simulink model "PVarray_Grid_IncCondReg_det"  (Simulink 10.0)
settings: Solver=FixedStepDiscrete  StartTime=0.0  StopTime=3  RelTol=1e-3
PreLoadFcn:
  | Ts_Power=1e-6
  | Ts_Control=100e-6
undefined symbols (not defined in the file): D1, Delta, DiscIntNeverNeededParam, level, sigbuilder_block
libraries: powerlib x29, powerlib_extras x7, simulink x4
(part 2 of 2)

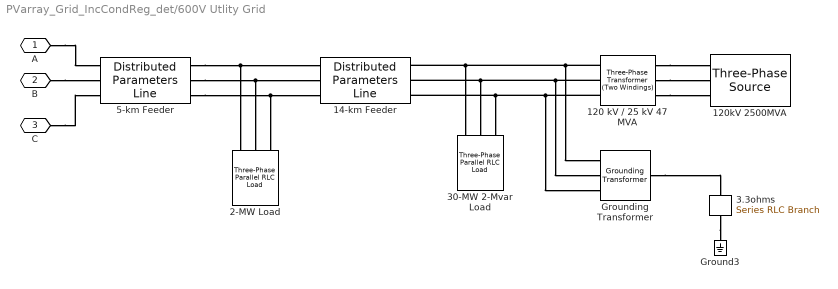
== system PVarray_Grid_IncCondReg_det/600V Utlity Grid ==
  120 kV / 25 kV 47 MVA : powerlib/Elements/Three-Phase Transformer (Two Windings)  Winding1Connection=Yg  Winding2Connection=Delta (D1)  CoreType=Three single-phase transformers  SetSaturation=off  Hysteresis=off  DataFile='basic_model'  SetInitialFlux=off  Measurements=None  UNITS=pu  NominalPower=[47e6 60 ]  Winding1="[ 120e3  0.08/30   0.08 ]"  Winding2="[ 25e3  0.08/30  0.08]"  Rm=500  Lm=500  L0=0.5  Saturation="[ 0,0  ;  0.005,1.2  ;  1.0,1.4 ]"  InitialFluxes=[ 0.8 , -0.8 , 0.7 ]  BreakLoop=off  DiscreteSolver=Trapezoidal iterative  DataType=off  TransfoNumber=0
      settings: SourceProductName=Simscape Electrical
  120kV 2500MVA : powerlib/Electrical Sources/Three-Phase Source  InternalConnection=Yg  VoltagePhases=off  Voltage=120e3  PhaseAngle=0  Voltage_phases=[25e3 25e3 25e3]/sqrt(3)  PhaseAngles_phases=[0 -120 +120]  Frequency=60  NonIdealSource=on  SpecifyImpedance=on  Resistance=0.8929  Inductance=16.58e-3  ShortCircuitLevel=2500e6  BaseVoltage=120e3  XRratio=7  BusType=swing  Pref=0  Qref=0  Prefabc=[10e3, 10e3, 10e3]  Qrefabc=[0, 0, 0]  Qmin=-inf  Qmax=inf
      settings: SourceProductName=Simscape Electrical
  14-km Feeder : powerlib/Elements/Distributed Parameters Line  Phases=3  Frequency=60  Resistance=[0.1153 0.413]  Inductance=[1.05e-3 3.32e-3]  Capacitance=[11.33e-009 5.01e-009]  Length=14  x1=[-5.8e-05 3.86893483226121e-09 0 0;-5.7e-05 3.86863781931287e-09 0 0;-5.6e-05 3.86834025654481e-09 0 0;-5.5e-05 3.86804214399933e-09 0 0;-5.4e-05 3.8677434817188e-09 0 0;-5.3e-05 3.86744426974566e-09 0 0;-5.2e-05 3.86714450812244e-09 0 0;-5.1e-05 3.86684419689175e-09 0 0;-5e-05 3.86654333609625e-09 0 0;-4.9e-05 3.86624192577872e-09 -3790.50088209685 -24060.9143986491;-4.8e-05 3.86593996598198e-09 -3781.42986192474 -24062.341673986;-4.7e-05 3.86563745674896e-09 -3772.35830432711 -24063.7655295274;-4.6e-05 3.86533439812265e-09 -3763.28621059323 -24065.1859650711;-4.5e-05 3.86503079014612e-09 -3754.21358201246 -24066.6029804152;-4.4e-05 3.86472663286251e-09 -3745.14041987422 -24068.0165753583;-4.3e-05 3.86442192631506e-09 -3736.06672546799 -24069.4267496995;-4.2e-05 3.86411667054707e-09 -3726.99250008337 -24070.8335032383;-4.1e-05 3.86381086560192e-09 -3717.91774500999 -24072.2368357749;-4e-05 3.86350451152308e-09 -3708.84246153758 -24073.6367471098;-3.9e-05 3.86319760835409e-09 -3699.76665095595 -24075.033237044;-3.8e-05 3.86289015613856e-09 -3690.69031455496 -24076.426305379;-3.7e-05 3.86258215492019e-09 -3681.61345362458 -24077.815951917;-3.6e-05 3.86227360474275e-09 -3672.53606945481 -24079.2021764603;-3.5e-05 3.8619645056501e-09 -3663.45816333577 -24080.584978812;-3.4e-05 3.86165485768617e-09 -3654.37973655762 -24081.9643587755;-3.3e-05 3.86134466089496e-09 -3645.30079041061 -24083.3403161549;-3.2e-05 3.86103391532056e-09 -3636.22132618506 -24084.7128507544;-3.1e-05 3.86072262100713e-09 -3627.14134517136 -24086.0819623792;-3e-05 3.86041077799891e-09 -3618.06084865999 -24087.4476508345;-2.9e-05 3.86009838634023e-09 -3608.97983794149 -24088.8099159263;-2.8e-05 3.85978544607549e-09 -3599.89831430646 -24090.168757461;-2.7e-05 3.85947195724915e-09 -3590.8162790456 -24091.5241752455;-2.6e-05 3.85915791990577e-09 -3581.73373344966 -24092.8761690871;-2.5e-05 3.85884333408999e-09 -3572.65067880949 -24094.2247387938;-2.4e-05 3.85852819984651e-09 -3563.56711641597 -24095.5698841737;-2.3e-05 3.85821251722012e-09 -3554.48304756009 -24096.9116050357;-2.2e-05 3.85789628625569e-09 -3545.39847353291 -24098.2499011893;-2.1e-05 3.85757950699816e-09 -3536.31339562553 -24099.5847724441;-2e-05 3.85726217949255e-09 -3527.22781512915 -24100.9162186104;-1.9e-05 3.85694430378396e-09 -3518.14173333503 -24102.244239499;-1.8e-05 3.85662587991757e-09 -3509.05515153452 -24103.5688349213;-1.7e-05 3.85630690793864e-09 -3499.96807101901 -24104.8900046888;-1.6e-05 3.85598738789248e-09 -3490.88049307998 -24106.2077486139;-1.5e-05 3.85566731982453e-09 -3481.79241900898 -24107.5220665093;-1.4e-05 3.85534670378026e-09 -3472.70385009763 -24108.8329581881;-1.3e-05 3.85502553980525e-09 -3463.61478763761 -24110.1404234641;-1.2e-05 3.85470382794513e-09 -3454.52523292069 -24111.4444621514;-1.1e-05 3.85438156824563e-09 -3445.43518723869 -24112.7450740648;-1e-05 3.85405876075255e-09 -3436.34465188351 -24114.0422590193;-9e-06 3.85373540551177e-09 -3427.25362814712 -24115.3360168307;-8e-06 3.85341150256924e-09 -3418.16211732156 -24116.626347315;-7e-06 3.853087051971e-09 -3409.07012069893 -24117.9132502888;-6e-06 3.85276205376316e-09 -3399.9776395714 -24119.1967255693;-5e-06 3.85243650799191e-09 -3390.88467523123 -24120.4767729741;-4e-06 3.85211041470352e-09 -3381.79122897072 -24121.7533923211;-3e-06 3.85178377394433e-09 -3372.69730208226 -24123.0265834291;-2e-06 3.85145658576076e-09 -3363.6028958583 -24124.296346117;-1e-06 3.85112885019932e-09 -3354.50801159135 -24125.5626802043]  x2=[-5.8e-05 4.13964869045981e-09 0 0;-5.7e-05 4.13926412209804e-09 0 0;-5.6e-05 4.13887896545453e-09 0 0;-5.5e-05 4.13849322058402e-09 0 0;-5.4e-05 4.13810688754132e-09 0 0;-5.3e-05 4.13771996638135e-09 0 0;-5.2e-05 4.1373324571591e-09 0 0;-5.1e-05 4.13694435992963e-09 0 0;-5e-05 4.13655567474811e-09 0 0;-4.9e-05 4.13616640166977e-09 -3379.33798533028 -24243.9018981742;-4.8e-05 4.13577654074994e-09 -3370.19800971541 -24245.1741557511;-4.7e-05 4.13538609204404e-09 -3361.05755512023 -24246.442967548;-4.6e-05 4.13499505560754e-09 -3351.91662284382 -24247.7083333847;-4.5e-05 4.13460343149603e-09 -3342.77521418531 -24248.9702530812;-4.4e-05 4.13421121976516e-09 -3333.63333044389 -24250.2287264583;-4.3e-05 4.13381842047068e-09 -3324.49097291882 -24251.4837533371;-4.2e-05 4.13342503366841e-09 -3315.34814290945 -24252.7353335391;-4.1e-05 4.13303105941426e-09 -3306.20484171517 -24253.9834668866;-4e-05 4.13263649776422e-09 -3297.06107063545 -24255.2281532022;-3.9e-05 4.13224134877437e-09 -3287.91683096981 -24256.4693923088;-3.8e-05 4.13184561250087e-09 -3278.77212401787 -24257.7071840303;-3.7e-05 4.13144928899996e-09 -3269.62695107929 -24258.9415281905;-3.6e-05 4.13105237832797e-09 -3260.4813134538 -24260.1724246142;-3.5e-05 4.13065488054131e-09 -3251.33521244121 -24261.3998731263;-3.4e-05 4.13025679569647e-09 -3242.18864934136 -24262.6238735524;-3.3e-05 4.12985812385002e-09 -3233.04162545421 -24263.8444257185;-3.2e-05 4.12945886505863e-09 -3223.89414207974 -24265.0615294512;-3.1e-05 4.12905901937905e-09 -3214.74620051801 -24266.2751845776;-3e-05 4.12865858686809e-09 -3205.59780206915 -24267.485390925;-2.9e-05 4.12825756758267e-09 -3196.44894803336 -24268.6921483216;-2.8e-05 4.12785596157979e-09 -3187.29963971088 -24269.8954565958;-2.7e-05 4.12745376891651e-09 -3178.14987840204 -24271.0953155766;-2.6e-05 4.12705098965e-09 -3168.99966540723 -24272.2917250934;-2.5e-05 4.12664762383751e-09 -3159.84900202689 -24273.4846849763;-2.4e-05 4.12624367153636e-09 -3150.69788956153 -24274.6741950557;-2.3e-05 4.12583913280396e-09 -3141.54632931174 -24275.8602551625;-2.2e-05 4.12543400769781e-09 -3132.39432257816 -24277.0428651282;-2.1e-05 4.12502829627548e-09 -3123.24187066148 -24278.2220247846;-2e-05 4.12462199859463e-09 -3114.08897486248 -24279.3977339643;-1.9e-05 4.12421511471301e-09 -3104.93563648199 -24280.5699925001;-1.8e-05 4.12380764468845e-09 -3095.7818568209 -24281.7388002254;-1.7e-05 4.12339958857886e-09 -3086.62763718016 -24282.904156974;-1.6e-05 4.12299094644222e-09 -3077.47297886081 -24284.0660625805;-1.5e-05 4.12258171833662e-09 -3068.3178831639 -24285.2245168796;-1.4e-05 4.12217190432022e-09 -3059.1623513906 -24286.3795197066;-1.3e-05 4.12176150445126e-09 -3050.00638484211 -24287.5310708975;-1.2e-05 4.12135051878806e-09 -3040.84998481968 -24288.6791702886;-1.1e-05 4.12093894738905e-09 -3031.69315262466 -24289.8238177168;-1e-05 4.1205267903127e-09 -3022.53588955843 -24290.9650130192;-9e-06 4.12011404761761e-09 -3013.37819692244 -24292.1027560338;-8e-06 4.11970071936242e-09 -3004.2200760182 -24293.2370465988;-7e-06 4.11928680560588e-09 -2995.0615281473 -24294.3678845531;-6e-06 4.11887230640683e-09 -2985.90255461135 -24295.4952697358;-5e-06 4.11845722182416e-09 -2976.74315671207 -24296.6192019869;-4e-06 4.11804155191686e-09 -2967.58333575119 -24297.7396811465;-3e-06 4.11762529674403e-09 -2958.42309303054 -24298.8567070555;-2e-06 4.11720845636481e-09 -2949.26242985199 -24299.970279555;-1e-06 4.11679103083845e-09 -2940.10134751747 -24301.0803984868]  x3=[-5.8e-05 2.1249422545882e-11 0 0;-5.7e-05 2.12530209427396e-11 0 0;-5.6e-05 2.1256616319069e-11 0 0;-5.5e-05 2.12602086743592e-11 0 0;-5.4e-05 2.12637980080996e-11 0 0;-5.3e-05 2.126738431978e-11 0 0;-5.2e-05 2.12709676088909e-11 0 0;-5.1e-05 2.12745478749228e-11 0 0;-5e-05 2.12781251173671e-11 0 0;-4.9e-05 2.12816993357152e-11 -23.610210034622 -155.666879550872;-4.8e-05 2.12852705294593e-11 -23.5515233272188 -155.675769328281;-4.7e-05 2.12888386980917e-11 -23.4928332726189 -155.684636980691;-4.6e-05 2.12924038411053e-11 -23.4341398791635 -155.693482506843;-4.5e-05 2.12959659579935e-11 -23.3754431551942 -155.702305905478;-4.4e-05 2.129952504825e-11 -23.3167431090532 -155.711107175343;-4.3e-05 2.1303081111369e-11 -23.2580397490829 -155.719886315187;-4.2e-05 2.13066341468451e-11 -23.1993330836265 -155.728643323763;-4.1e-05 2.13101841541732e-11 -23.1406231210274 -155.737378199825;-4e-05 2.1313731132849e-11 -23.0819098696298 -155.746090942133;-3.9e-05 2.13172750823682e-11 -23.023193337778 -155.754781549447;-3.8e-05 2.13208160022272e-11 -22.9644735338169 -155.763450020534;-3.7e-05 2.13243538919228e-11 -22.9057504660921 -155.772096354161;-3.6e-05 2.13278887509522e-11 -22.8470241429492 -155.780720549098;-3.5e-05 2.13314205788128e-11 -22.7882945727347 -155.789322604122;-3.4e-05 2.13349493750029e-11 -22.7295617637953 -155.797902518008;-3.3e-05 2.13384751390209e-11 -22.6708257244783 -155.806460289537;-3.2e-05 2.13419978703657e-11 -22.6120864631313 -155.814995917494;-3.1e-05 2.13455175685366e-11 -22.5533439881026 -155.823509400665;-3e-05 2.13490342330335e-11 -22.4945983077407 -155.83200073784;-2.9e-05 2.13525478633564e-11 -22.4358494303947 -155.840469927813;-2.8e-05 2.13560584590061e-11 -22.3770973644142 -155.848916969379;-2.7e-05 2.13595660194836e-11 -22.318342118149 -155.857341861338;-2.6e-05 2.13630705442905e-11 -22.2595836999498 -155.865744602493;-2.5e-05 2.13665720329285e-11 -22.2008221181672 -155.87412519165;-2.4e-05 2.13700704849002e-11 -22.1420573811527 -155.882483627618;-2.3e-05 2.13735658997083e-11 -22.0832894972581 -155.890819909208;-2.2e-05 2.1377058276856e-11 -22.0245184748355 -155.899134035236;-2.1e-05 2.13805476158469e-11 -21.9657443222377 -155.90742600452;-2e-05 2.13840339161853e-11 -21.9069670478177 -155.915695815882;-1.9e-05 2.13875171773755e-11 -21.8481866599292 -155.923943468146;-1.8e-05 2.13909973989225e-11 -21.789403166926 -155.932168960141;-1.7e-05 2.13944745803318e-11 -21.7306165771628 -155.940372290697;-1.6e-05 2.1397948721109e-11 -21.6718268989943 -155.948553458648;-1.5e-05 2.14014198207606e-11 -21.6130341407758 -155.956712462832;-1.4e-05 2.14048878787931e-11 -21.5542383108633 -155.964849302089;-1.3e-05 2.14083528947137e-11 -21.4954394176127 -155.972963975263;-1.2e-05 2.14118148680299e-11 -21.4366374693808 -155.981056481199;-1.1e-05 2.14152737982497e-11 -21.3778324745247 -155.98912681875;-1e-05 2.14187296848815e-11 -21.3190244414018 -155.997174986766;-9e-06 2.14221825274341e-11 -21.2602133783701 -156.005200984105;-8e-06 2.14256323254168e-11 -21.2013992937879 -156.013204809626;-7e-06 2.14290790783393e-11 -21.1425821960141 -156.02118646219;-6e-06 2.14325227857118e-11 -21.0837620934078 -156.029145940665;-5e-06 2.14359634470449e-11 -21.0249389943287 -156.037083243919;-4e-06 2.14394010618494e-11 -20.9661129071369 -156.044998370822;-3e-06 2.1442835629637e-11 -20.9072838401929 -156.052891320252;-2e-06 2.14462671499194e-11 -20.8484518018576 -156.060762091086;-1e-06 2.14496956222089e-11 -20.7896168004923 -156.068610682204]  x4=[-5.8e-05 -1.15723579337896e-11 0 0;-5.7e-05 -1.15764232992851e-11 0 0;-5.6e-05 -1.15804870195128e-11 0 0;-5.5e-05 -1.1584549093895e-11 0 0;-5.4e-05 -1.15886095218544e-11 0 0;-5.3e-05 -1.15926683028139e-11 0 0;-5.2e-05 -1.15967254361968e-11 0 0;-5.1e-05 -1.16007809214263e-11 0 0;-5e-05 -1.16048347579262e-11 0 0;-4.9e-05 -1.16088869451202e-11 -1.28892375629152 -2.16547060902535;-4.8e-05 -1.16129374824325e-11 -1.28810730153162 -2.16595636794147;-4.7e-05 -1.16169863692873e-11 -1.28729066370296 -2.16644181902688;-4.6e-05 -1.16210336051094e-11 -1.28647384292158 -2.16692696221259;-4.5e-05 -1.16250791893234e-11 -1.28565683930357 -2.16741179742966;-4.4e-05 -1.16291231213544e-11 -1.28483965296506 -2.16789632460917;-4.3e-05 -1.16331654006276e-11 -1.28402228402218 -2.16838054368227;-4.2e-05 -1.16372060265686e-11 -1.28320473259109 -2.16886445458013;-4.1e-05 -1.16412449986031e-11 -1.282386998788 -2.16934805723399;-4e-05 -1.1645282316157e-11 -1.28156908272911 -2.1698313515751;-3.9e-05 -1.16493179786567e-11 -1.28075098453068 -2.17031433753479;-3.8e-05 -1.16533519855284e-11 -1.27993270430896 -2.17079701504441;-3.7e-05 -1.1657384336199e-11 -1.27911424218027 -2.17127938403536;-3.6e-05 -1.16614150300952e-11 -1.27829559826092 -2.17176144443909;-3.5e-05 -1.16654440666443e-11 -1.27747677266725 -2.17224319618709;-3.4e-05 -1.16694714452737e-11 -1.27665776551564 -2.17272463921088;-3.3e-05 -1.16734971654109e-11 -1.2758385769225 -2.17320577344204;-3.2e-05 -1.16775212264838e-11 -1.27501920700423 -2.1736865988122;-3.1e-05 -1.16815436279205e-11 -1.27419965587731 -2.17416711525301;-3e-05 -1.16855643691493e-11 -1.27337992365819 -2.17464732269619;-2.9e-05 -1.16895834495989e-11 -1.27256001046339 -2.17512722107349;-2.8e-05 -1.16936008686979e-11 -1.27173991640944 -2.1756068103167;-2.7e-05 -1.16976166258755e-11 -1.27091964161288 -2.17608609035766;-2.6e-05 -1.17016307205609e-11 -1.27009918619029 -2.17656506112826;-2.5e-05 -1.17056431521835e-11 -1.26927855025828 -2.17704372256042;-2.4e-05 -1.17096539201733e-11 -1.26845773393349 -2.17752207458612;-2.3e-05 -1.171366302396e-11 -1.26763673733256 -2.17800011713737;-2.2e-05 -1.17176704629741e-11 -1.26681556057218 -2.17847785014623;-2.1e-05 -1.17216762366458e-11 -1.26599420376906 -2.1789552735448;-2e-05 -1.17256803444059e-11 -1.26517266703993 -2.17943238726523;-1.9e-05 -1.17296827856853e-11 -1.26435095050155 -2.17990919123972;-1.8e-05 -1.17336835599152e-11 -1.2635290542707 -2.18038568540049;-1.7e-05 -1.1737682666527e-11 -1.26270697846419 -2.18086186967984;-1.6e-05 -1.17416801049524e-11 -1.26188472319886 -2.18133774401007;-1.5e-05 -1.17456758746231e-11 -1.26106228859157 -2.18181330832356;-1.4e-05 -1.17496699749713e-11 -1.2602396747592 -2.18228856255273;-1.3e-05 -1.17536624054294e-11 -1.25941688181867 -2.18276350663002;-1.2e-05 -1.17576531654299e-11 -1.25859390988691 -2.18323814048793;-1.1e-05 -1.17616422544057e-11 -1.25777075908089 -2.18371246405902;-1e-05 -1.17656296717899e-11 -1.2569474295176 -2.18418647727587;-9e-06 -1.17696154170156e-11 -1.25612392131404 -2.1846601800711;-8e-06 -1.17735994895166e-11 -1.25530023458726 -2.18513357237741;-7e-06 -1.17775818887265e-11 -1.25447636945433 -2.18560665412749;-6e-06 -1.17815626140793e-11 -1.25365232603232 -2.18607942525414;-5e-06 -1.17855416650093e-11 -1.25282810443836 -2.18655188569014;-4e-06 -1.1789519040951e-11 -1.25200370478958 -2.18702403536835;-3e-06 -1.17934947413392e-11 -1.25117912720316 -2.18749587422168;-2e-06 -1.17974687656087e-11 -1.25035437179628 -2.18796740218306;-1e-06 -1.18014411131948e-11 -1.24952943868616 -2.18843861918547]  x5=5.70973484498186e-05  V1=ones(3,3)  V2=ones(3,3)  I1=ones(3,3)  I2=ones(3,3)  nHarmo=1  Measurements=None
      settings: SourceProductName=Simscape Electrical
  2-MW Load : powerlib/Elements/Three-Phase Parallel RLC Load  LConnTagsString=A|B|C  Configuration=Y (grounded)  NominalVoltage=25e3  Vabc=[1e3 1e3 1e3]  Vabcp=[1e3 1e3 1e3]  NominalFrequency=60  UnbalancedPower=off  ActivePower=2e6  InductivePower=0  CapacitivePower=0  Pabc=[10e3 9e3 11e3]  QLabc=[100 90 110]  QCabc=[100 90 110]  Pabcp=[10e3 9e3 11e3]  QLabcp=[100 90 110]  QCabcp=[100 90 110]  Measurements=None  LoadType=constant Z
      settings: SourceProductName=Simscape Electrical
  "3.3ohms " : powerlib/Elements/Series RLC Branch  LConnTagsString=__new0  RConnTagsString=__new0  BranchType=R  Resistance=3.3  Inductance=[]  SetiL0=off  InitialCurrent=0  Capacitance=[]  Setx0=off  InitialVoltage=0  Measurements=None
      settings: SourceProductName=Simscape Electrical
  30-MW 2-Mvar Load : powerlib/Elements/Three-Phase Parallel RLC Load  LConnTagsString=A|B|C  Configuration=Y (grounded)  NominalVoltage=25e3  Vabc=[1e3 1e3 1e3]  Vabcp=[1e3 1e3 1e3]  NominalFrequency=60  UnbalancedPower=off  ActivePower=30e6  InductivePower=2e6  CapacitivePower=0  Pabc=[10e3 9e3 11e3]  QLabc=[100 90 110]  QCabc=[100 90 110]  Pabcp=[10e3 9e3 11e3]  QLabcp=[100 90 110]  QCabcp=[100 90 110]  Measurements=None  LoadType=constant Z
      settings: SourceProductName=Simscape Electrical
  5-km Feeder : powerlib/Elements/Distributed Parameters Line  Phases=3  Frequency=60  Resistance=[0.1153 0.413]  Inductance=[1.05e-3 3.32e-3]  Capacitance=[11.33e-009 5.01e-009]  Length=5  x1=[-2.1e-05 3.77032655351987e-09 -3536.8883456393 -24100.782456775;-2e-05 3.77000631445996e-09 -3527.80231358572 -24102.1141196072;-1.9e-05 3.76968553959807e-09 -3518.71578015276 -24103.4423569916;-1.8e-05 3.76936422897981e-09 -3509.6287466318 -24104.7671687392;-1.7e-05 3.76904238265082e-09 -3500.54121431434 -24106.0885546618;-1.6e-05 3.76872000065685e-09 -3491.4531844919 -24107.4065145717;-1.5e-05 3.76839708304372e-09 -3482.36465845609 -24108.7210482814;-1.4e-05 3.76807362985732e-09 -3473.27563749861 -24110.0321556042;-1.3e-05 3.76774964114363e-09 -3464.1861229112 -24111.3398363538;-1.2e-05 3.76742511694869e-09 -3455.09611598568 -24112.6440903442;-1.1e-05 3.76710005731861e-09 -3446.00561801395 -24113.9449173902;-1e-05 3.76677446229961e-09 -3436.91463028797 -24115.2423173068;-9e-06 3.76644833193795e-09 -3427.82315409977 -24116.5362899096;-8e-06 3.76612166627998e-09 -3418.73119074146 -24117.8268350149;-7e-06 3.76579446537214e-09 -3409.6387415052 -24119.113952439;-6e-06 3.76546672926091e-09 -3400.54580768323 -24120.3976419992;-5e-06 3.76513845799289e-09 -3391.45239056787 -24121.6779035129;-4e-06 3.76480965161472e-09 -3382.35849145148 -24122.9547367983;-3e-06 3.76448031017315e-09 -3373.26411162652 -24124.2281416738;-2e-06 3.76415043371496e-09 -3364.16925238551 -24125.4981179584;-1e-06 3.76382002228705e-09 -3355.07391502101 -24126.7646654718]  x2=[-2.1e-05 3.85848717314219e-09 -3536.31339562553 -24099.5847724441;-2e-05 3.85816993400167e-09 -3527.22781512915 -24100.9162186104;-1.9e-05 3.85785214652916e-09 -3518.14173333503 -24102.244239499;-1.8e-05 3.85753381076982e-09 -3509.05515153452 -24103.5688349213;-1.7e-05 3.8572149267689e-09 -3499.96807101901 -24104.8900046888;-1.6e-05 3.85689549457171e-09 -3490.88049307998 -24106.2077486139;-1.5e-05 3.85657551422366e-09 -3481.79241900898 -24107.5220665093;-1.4e-05 3.85625498577022e-09 -3472.70385009763 -24108.8329581881;-1.3e-05 3.85593390925695e-09 -3463.61478763761 -24110.1404234641;-1.2e-05 3.85561228472947e-09 -3454.52523292069 -24111.4444621514;-1.1e-05 3.8552901122335e-09 -3445.43518723869 -24112.7450740648;-1e-05 3.85496739181483e-09 -3436.34465188351 -24114.0422590193;-9e-06 3.85464412351931e-09 -3427.25362814712 -24115.3360168307;-8e-06 3.85432030739291e-09 -3418.16211732156 -24116.626347315;-7e-06 3.85399594348162e-09 -3409.07012069893 -24117.9132502888;-6e-06 3.85367103183157e-09 -3399.9776395714 -24119.1967255693;-5e-06 3.85334557248892e-09 -3390.88467523123 -24120.4767729741;-4e-06 3.85301956549992e-09 -3381.79122897072 -24121.7533923211;-3e-06 3.85269301091092e-09 -3372.69730208226 -24123.0265834291;-2e-06 3.85236590876832e-09 -3363.6028958583 -24124.296346117;-1e-06 3.85203825911861e-09 -3354.50801159135 -24125.5626802043]  x3=[-2.1e-05 8.43243860018511e-12 -11.2236902755189 -79.1234381044604;-2e-05 8.43641569553715e-12 -11.193860645232 -79.1276637133075;-1.9e-05 8.44039159188637e-12 -11.1640294240479 -79.1318780763489;-1.8e-05 8.44436628866772e-12 -11.1341966162062 -79.1360811929856;-1.7e-05 8.44833978531629e-12 -11.1043622259469 -79.1402730626204;-1.6e-05 8.45231208126737e-12 -11.07452625751 -79.1444536846574;-1.5e-05 8.4562831759564e-12 -11.044688715136 -79.1486230585024;-1.4e-05 8.46025306881899e-12 -11.0148496030654 -79.152781183563;-1.3e-05 8.46422175929096e-12 -10.985008925539 -79.1569280592481;-1.2e-05 8.46818924680824e-12 -10.9551666867979 -79.1610636849684;-1.1e-05 8.47215553080697e-12 -10.9253228910833 -79.1651880601362;-1e-05 8.47612061072346e-12 -10.8954775426366 -79.1693011841652;-9e-06 8.48008448599418e-12 -10.8656306456996 -79.1734030564709;-8e-06 8.48404715605578e-12 -10.8357822045141 -79.1774936764703;-7e-06 8.48800862034506e-12 -10.8059322233224 -79.1815730435821;-6e-06 8.49196887829902e-12 -10.7760807063666 -79.1856411572264;-5e-06 8.49592792935482e-12 -10.7462276578895 -79.1896980168252;-4e-06 8.49988577294979e-12 -10.7163730821338 -79.1937436218018;-3e-06 8.50384240852143e-12 -10.6865169833425 -79.1977779715813;-2e-06 8.50779783550741e-12 -10.6566593657588 -79.2018010655904;-1e-06 8.51175205334558e-12 -10.6268002336261 -79.2058129032571]  x4=[-2.1e-05 9.67844381521477e-13 -12.4922083172284 -78.9091123636644;-2e-05 9.62308848136267e-13 -12.462459395698 -78.9138162077657;-1.9e-05 9.56773177985509e-13 -12.4327087029741 -78.9185088364538;-1.8e-05 9.51237371855945e-13 -12.4029562432851 -78.9231902490618;-1.7e-05 9.45701430534336e-13 -12.3732020208594 -78.9278604449243;-1.6e-05 9.40165354807463e-13 -12.3434460399258 -78.9325194233777;-1.5e-05 9.34629145462125e-13 -12.3136883047131 -78.9371671837597;-1.4e-05 9.29092803285143e-13 -12.2839288194508 -78.9418037254098;-1.3e-05 9.23556329063352e-13 -12.2541675883682 -78.946429047669;-1.2e-05 9.18019723583611e-13 -12.2244046156951 -78.9510431498801;-1.1e-05 9.12482987632793e-13 -12.1946399056615 -78.9556460313871;-1e-05 9.06946121997793e-13 -12.1648734624976 -78.9602376915361;-9e-06 9.01409127465523e-13 -12.1351052904339 -78.9648181296743;-8e-06 8.95872004822912e-13 -12.1053353937011 -78.9693873451508;-7e-06 8.9033475485691e-13 -12.0755637765302 -78.9739453373162;-6e-06 8.84797378354484e-13 -12.0457904431523 -78.9784921055227;-5e-06 8.79259876102618e-13 -12.016015397799 -78.9830276491242;-4e-06 8.73722248888314e-13 -11.9862386447019 -78.9875519674759;-3e-06 8.68184497498593e-13 -11.956460188093 -78.992065059935;-2e-06 8.62646622720493e-13 -11.9266800322045 -78.99656692586;-1e-06 8.5710862534107e-13 -11.8968981812687 -79.001057564611]  x5=2.03919101606495e-05  V1=ones(3,3)  V2=ones(3,3)  I1=ones(3,3)  I2=ones(3,3)  nHarmo=1  Measurements=None
      settings: SourceProductName=Simscape Electrical
  Ground3 : powerlib/Elements/Ground  LConnTagsString=a
      settings: SourceProductName=Simscape Electrical
  "Grounding Transformer " : powerlib/Elements/Grounding Transformer   UNITS=pu  NominalPower="[100e6   60]"  NominalVoltage=25e3  ZeroSequenceImpedance_pu=[0.025 0.75]  MagnetizationBranch_pu=[500 500]  ZeroSequenceImpedance_SI=[0.052083 589.05]  MagnetizationBranch_SI=[1041.7 3.927e+005]  Measurements=None
      settings: SourceProductName=Simscape Electrical  SourceProductBaseCode=PS
  A : PMIOPort  Side=Left
  B : PMIOPort  Port=2  Side=Left
  C : PMIOPort  Port=3  Side=Left
  connections:
  "3.3ohms "/RConn1 -- Ground3/LConn1
  120 kV / 25 kV 47 MVA/LConn1 -- 120kV 2500MVA/RConn1
  120 kV / 25 kV 47 MVA/LConn2 -- 120kV 2500MVA/RConn2
  120 kV / 25 kV 47 MVA/LConn3 -- 120kV 2500MVA/RConn3
  120 kV / 25 kV 47 MVA/RConn1 -- "Grounding Transformer "/LConn1 -- 14-km Feeder/RConn1 -- 30-MW 2-Mvar Load/LConn1
  120 kV / 25 kV 47 MVA/RConn2 -- "Grounding Transformer "/LConn2 -- 14-km Feeder/RConn2 -- 30-MW 2-Mvar Load/LConn2
  120 kV / 25 kV 47 MVA/RConn3 -- "Grounding Transformer "/LConn3 -- 14-km Feeder/RConn3 -- 30-MW 2-Mvar Load/LConn3
  5-km Feeder/RConn1 -- 14-km Feeder/LConn1 -- 2-MW Load/LConn1
  5-km Feeder/RConn2 -- 14-km Feeder/LConn2 -- 2-MW Load/LConn2
  5-km Feeder/RConn3 -- 14-km Feeder/LConn3 -- 2-MW Load/LConn3
  A/RConn1 -- 5-km Feeder/LConn1
  B/RConn1 -- 5-km Feeder/LConn2
  C/RConn1 -- 5-km Feeder/LConn3
  "Grounding Transformer "/RConn1 -- "3.3ohms "/LConn1

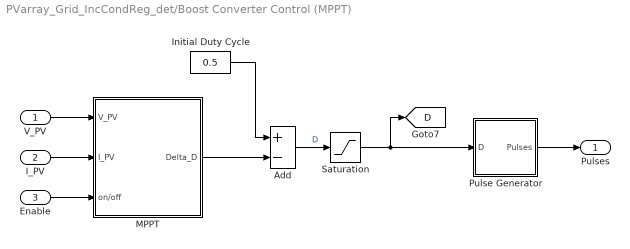
== system PVarray_Grid_IncCondReg_det/Boost Converter Control (MPPT) ==
  V_PV : Inport
  I_PV : Inport  Port=2
  Enable : Inport  Port=3
  Add : Sum  Inputs=+-
  Initial Duty Cycle : Constant  Value=0.5
  MPPT : Subsystem
  Pulse Generator : Subsystem  mask{Freq=5000}
      mask prompts: Freq "Frequency (Hz)"
  Saturation : Saturate  UpperLimit=1  LowerLimit=0
  Pulses : Outport
  tag scope: D=global
  wires:
  Initial Duty Cycle/1 -> Add/1
  MPPT/1(Delta_D) -> Add/2
  Add/1 -> Saturation/1  "D"
  Saturation/1 -> Pulse Generator/1(D), [D]
  Enable/1 -> MPPT/3(on/off)
  Pulse Generator/1(Pulses) -> Pulses/1
  I_PV/1 -> MPPT/2(I_PV)
  V_PV/1 -> MPPT/1(V_PV)

== system PVarray_Grid_IncCondReg_det/Irradiance (W/m2)  ==
  Demux : Demux  Tag=STV Demux  Outputs=1
  FromWs : FromWorkspace  Tag=STV FromWs  VariableName=tuvar  SampleTime=0  SigBuilderData=DataTag0  VnvData=DataTag1
      SigBuilderData=|
      | common.afterFinalStr = 'Extrapolate'
      | common.sampleTime = '0'
      | dataSet(1).timeRange = [0 1]
      | dataSet(1).name = 'Constant Irradiance'
      | dataSet(2).timeRange = [0 1]
      | dataSet(2).name = 'Step Irradiance'
      | dataSet(3).timeRange = [0 3]
      | dataSet(3).name = 'Ramp-up/down Irradiance'
      | sbobj.Groups(1).Name = 'Constant Irradiance'
      | sbobj.Groups(1).Signals.Name = 'Ir'
      | sbobj.Groups(1).Signals.XData = [0 1]
      | sbobj.Groups(1).Signals.YData = [1000 1000]
      | sbobj.Groups(1).TimeRange = [0 1]
      | sbobj.Groups(2).Name = 'Step Irradiance'
      | sbobj.Groups(2).Signals.Name = 'Ir'
      | sbobj.Groups(2).Signals.XData = [0 0.501 0.51 0.69 0.7 1]
      | sbobj.Groups(2).Signals.YData = [1000 1000 250 250 1000 1000]
      | sbobj.Groups(2).TimeRange = [0 1]
      | sbobj.Groups(3).Name = 'Ramp-up/down Irradiance'
      | sbobj.Groups(3).Signals.Name = 'Ir'
      | sbobj.Groups(3).Signals.XData = [0 0.7 1.2 1.5 2 2.3 2.35 2.65 2.7 3]
      | sbobj.Groups(3).Signals.YData = [1000 1000 250 250 1000 1000 250 250 1000 1000]
      | sbobj.Groups(3).TimeRange = [0 3]
  Ir : Outport  Tag=STV Outport
  wires:
  Demux/1 -> Ir/1
  FromWs/1 -> Demux/1

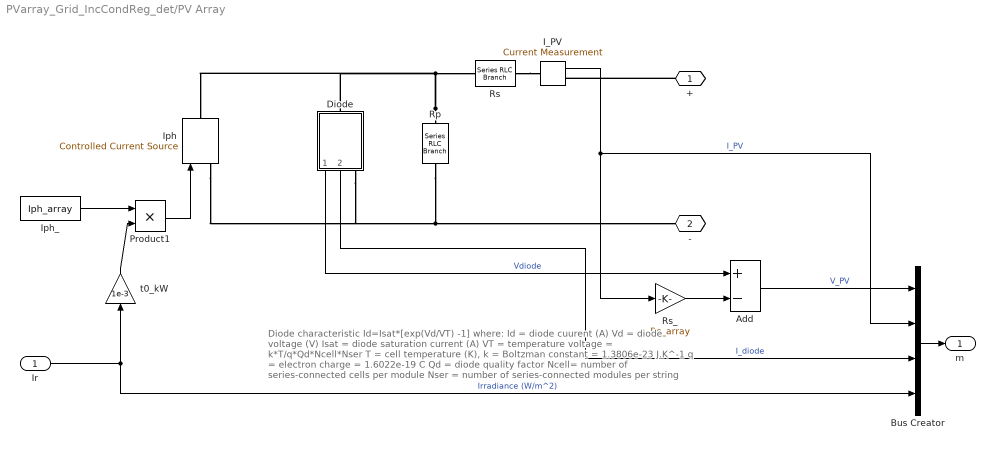
== system PVarray_Grid_IncCondReg_det/PV Array ==
  note: Diode characteristic
      |    Id=Isat*[exp(Vd/VT) -1]
      |
      | where:
      |    Id = diode cuurent (A)
      |    Vd = diode voltage (V)
      |  Isat = diode saturation current (A)
      |    VT = temperature voltage = k*T/q*Qd*Ncell*Nser
      |
      |     T = cell temperature (K),
      |     k = Boltzman constant = 1.3806e-23 J.K^-1
      |     q = electron charge = 1.6022e-19 C
      |    Qd = diode quality factor
      |  Ncell= number of series-connected cells per module
      |  Nser = number of series-connected modules per string
  Ir : Inport
  Add : Sum  Inputs=+-
  Bus Creator : BusCreator  Inputs=4
  Diode : Subsystem
      mask Display:
      | plot(-75,-50,100,150, [-15 -15 43 -15 -15 -75],[50 8 50 92 50 50], ...
      |     [43 43],[8 94],[100 43], [50 50])
  I_PV : powerlib/Measurements/Current Measurement  PhasorSimulation=off  OutputType=Complex  PSBequivalent=0
      settings: SourceProductName=Simscape Electrical
  Iph : powerlib/Electrical Sources/Controlled Current Source  Initialize=on  Source_Type=AC  Amplitude=0  Phase=0  Frequency=0  Measurements=None
      settings: SourceProductName=Simscape Electrical
  Iph_ : Constant  Value=Iph_array
  Product1 : Product  Inputs=**  RndMeth=Zero
  Rp : powerlib/Elements/Series RLC Branch  LConnTagsString=__new0  RConnTagsString=__new0  BranchType=R  Resistance=Rp_array  Inductance=1e-3  SetiL0=off  InitialCurrent=0  Capacitance=1e-6  Setx0=off  InitialVoltage=0  Measurements=Branch current
      settings: SourceProductName=Simscape Electrical
  Rs : powerlib/Elements/Series RLC Branch  LConnTagsString=__new0  RConnTagsString=__new0  BranchType=R  Resistance=Rs_array  Inductance=1e-3  SetiL0=off  InitialCurrent=0  Capacitance=1e-6  Setx0=off  InitialVoltage=0  Measurements=None
      settings: SourceProductName=Simscape Electrical
  Rs_ : Gain  Gain=Rs_array
  t0_kW : Gain  Gain=1e-3
  + : PMIOPort  Side=Right
  - : PMIOPort  Port=2  Side=Right
  m : Outport
  wires:
  Bus Creator/1 -> m/1
  Diode/2(Idiode) -> Bus Creator/3  "I_diode"
  Add/1 -> Bus Creator/1  "V_PV"
  t0_kW/1 -> Product1/2
  I_PV/1 -> Bus Creator/2, Rs_/1  "I_PV"
  Rs_/1 -> Add/2
  Diode/1(Vdiode) -> Add/1  "Vdiode"
  Ir/1 -> Bus Creator/4, t0_kW/1  "Irradiance (W/m^2)"
  Iph_/1 -> Product1/1
  Product1/1 -> Iph/1
  connections:
  +/RConn1 -- I_PV/RConn1
  Rs/LConn1 -- I_PV/LConn1
  Rp/LConn1 -- Rs/RConn1 -- Iph/RConn1 -- Diode/LConn1
  Rp/RConn1 -- -/RConn1 -- Diode/RConn1 -- Iph/LConn1

== system PVarray_Grid_IncCondReg_det/Pmean ==
  Discrete  Mean value : powerlib_extras/Discrete Measurements/Discrete  Mean value  Freq=60  Vinit=0  Ts=Ts_Control
      settings: SourceProductName=Simscape Electrical  SourceProductBaseCode=PS
  Product : Product  RndMeth=Zero
  WkW : Gain  Gain=1/1000
  V : Outport
  P : Outport  Port=2
  wires:
  [V_PV] -> Product/1, V/1
  Product/1 -> Discrete  Mean value/1
  [I_PV] -> Product/2
  WkW/1 -> P/1  "Pmean_PV (kW)"
  Discrete  Mean value/1 -> WkW/1

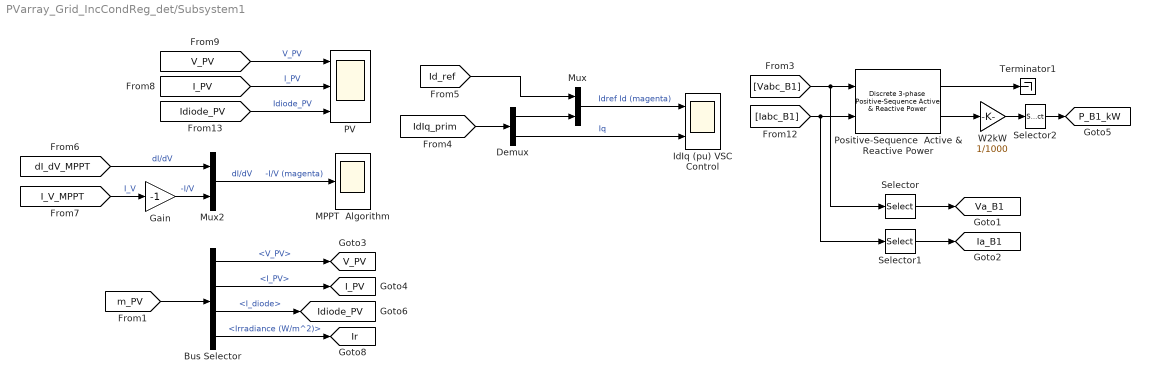
== system PVarray_Grid_IncCondReg_det/Subsystem1 ==
  Bus Selector : BusSelector  OutputSignals=V_PV,I_PV,I_diode,Irradiance (W/m^2)
  Demux : Demux  Outputs=2
  Gain : Gain  Gain=-1
  IdIq (pu) VSC Control : Scope  NumInputPorts=2
  MPPT  Algorithm : Scope
  Mux : Mux  Inputs=2
  Mux2 : Mux  Inputs=2
  PV : Scope  NumInputPorts=3
  Positive-Sequence  Active & Reactive Power : powerlib_extras/Discrete Measurements/Discrete 3-phase  Positive-Sequence  Active & Reactive Power  Freq=60  Par_Vinit=[0 0]  Par_Iinit=[0 0]  Ts=Ts_Control
      settings: SourceProductName=Simscape Electrical  SourceProductBaseCode=PS
  Selector : Selector  InputPortWidth=3  IndexOptions=Index vector (dialog)  Indices=[1]  OutputSizes=1
  Selector1 : Selector  InputPortWidth=3  IndexOptions=Index vector (dialog)  Indices=[1]  OutputSizes=1
  Selector2 : Selector  InputPortWidth=2  IndexOptions=Index vector (dialog)  Indices=[1]  OutputSizes=1
  Terminator1 : Terminator
  W2kW : Gain  Gain=1/1000
  tag scope: I_PV=global, Ia_B1=global, Idiode_PV=global, Ir=global, P_B1_kW=global, V_PV=global, Va_B1=global
  wires:
  [Vabc_B1] -> Positive-Sequence  Active & Reactive Power/1, Selector/1
  [Iabc_B1] -> Positive-Sequence  Active & Reactive Power/2, Selector1/1
  Positive-Sequence  Active & Reactive Power/2 -> W2kW/1
  Positive-Sequence  Active & Reactive Power/1 -> Terminator1/1
  W2kW/1 -> Selector2/1
  [I_V_MPPT] -> Gain/1  "I_V"
  [IdIq_prim] -> Demux/1
  [Id_ref] -> Mux/1
  Demux/1 -> Mux/2
  Mux/1 -> IdIq (pu) VSC Control/1  "Idref Id (magenta)"
  Demux/2 -> IdIq (pu) VSC Control/2  "Iq"
  Selector/1 -> [Va_B1]
  Selector1/1 -> [Ia_B1]
  [V_PV] -> PV/1  "V_PV"
  [I_PV] -> PV/2  "I_PV"
  [Idiode_PV] -> PV/3  "Idiode_PV"
  [dI_dV_MPPT] -> Mux2/1  "dI/dV"
  Gain/1 -> Mux2/2  "-I/V"
  Mux2/1 -> MPPT  Algorithm/1  "dI/dV     -I/V (magenta)"
  Selector2/1 -> [P_B1_kW]
  [m_PV] -> Bus Selector/1
  Bus Selector/1 -> [V_PV]  "<V_PV>"
  Bus Selector/2 -> [I_PV]  "<I_PV>"
  Bus Selector/3 -> [Idiode_PV]  "<I_diode>"
  Bus Selector/4 -> [Ir]  "<Irradiance (W/m^2)>"

== system PVarray_Grid_IncCondReg_det/Subsystem2 ==
  Discrete  Mean value : powerlib_extras/Discrete Measurements/Discrete  Mean value  Freq=60  Vinit=0  Ts=Ts_Control
      settings: SourceProductName=Simscape Electrical  SourceProductBaseCode=PS
  Mux1 : Mux  Inputs=2
  Vm : Outport
  "Vdc " : Outport  Port=2
  wires:
  [Vdc_ref] -> Mux1/1  "Vdc ref"
  [Vdc] -> Discrete  Mean value/1  "Vdc"
  Mux1/1 -> "Vdc "/1
  Discrete  Mean value/1 -> Mux1/2, Vm/1

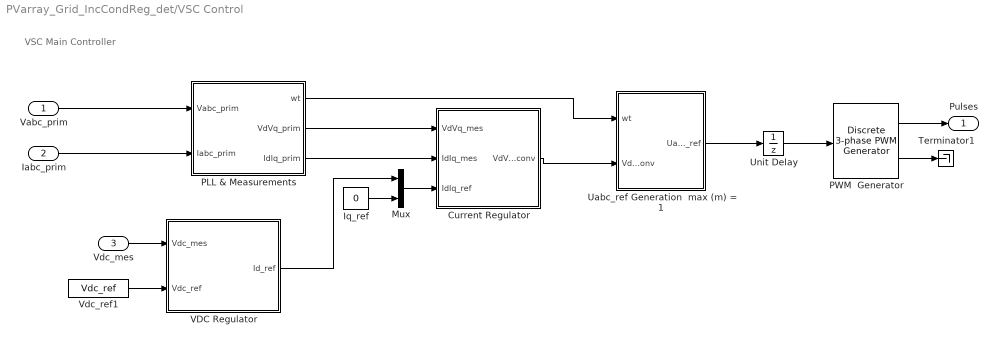
== system PVarray_Grid_IncCondReg_det/VSC Control ==
  note: VSC Main Controller
  Vabc_prim : Inport  PortDimensions=3
  Iabc_prim : Inport  Port=2  PortDimensions=3
  Vdc_mes : Inport  Port=3  PortDimensions=1
  Current Regulator : Subsystem
  Iq_ref : Constant  Value=0
  Mux : Mux  Inputs=2
  PLL & Measurements : Subsystem
  PWM  Generator : powerlib_extras/Discrete  Control Blocks/Discrete 3-phase PWM Generator  ModulatorType=3-level  ModulatorMode=Un-synchronized  nF=18  Fc=33*60  ModulatingSignals=off  m=0.2  Freq=60  Phase=0  Ts=Ts_Power
      settings: SourceProductName=Simscape Electrical  SourceProductBaseCode=PS
  Terminator1 : Terminator
  Uabc_ref Generation  max (m) = 1 : Subsystem
  Unit Delay : UnitDelay  SampleTime=Ts_Control  HasFrameUpgradeWarning=on
  VDC Regulator : Subsystem
  Vdc_ref1 : Constant  Value=Vdc_ref
  Pulses : Outport
  wires:
  VDC Regulator/1(Id_ref) -> Mux/1
  PLL & Measurements/1(wt) -> Uabc_ref Generation  max (m) = 1/1(wt)
  Current Regulator/1(VdVq_conv) -> Uabc_ref Generation  max (m) = 1/2(VdVq_conv)
  Iq_ref/1 -> Mux/2
  Mux/1 -> Current Regulator/3(IdIq_ref)
  PLL & Measurements/3(IdIq_prim) -> Current Regulator/2(IdIq_mes)
  PLL & Measurements/2(VdVq_prim) -> Current Regulator/1(VdVq_mes)
  Vdc_mes/1 -> VDC Regulator/1(Vdc_mes)
  Vabc_prim/1 -> PLL & Measurements/1(Vabc_prim)
  Iabc_prim/1 -> PLL & Measurements/2(Iabc_prim)
  Unit Delay/1 -> PWM  Generator/1
  PWM  Generator/1 -> Pulses/1
  Uabc_ref Generation  max (m) = 1/1(Uabc_ref) -> Unit Delay/1
  PWM  Generator/2 -> Terminator1/1
  Vdc_ref1/1 -> VDC Regulator/2(Vdc_ref)

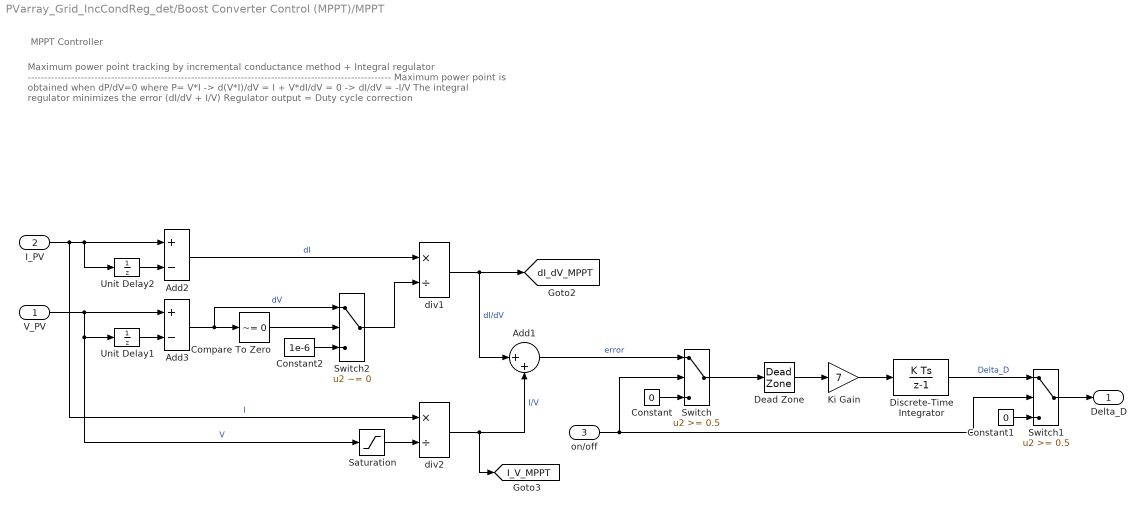
== system PVarray_Grid_IncCondReg_det/Boost Converter Control (MPPT)/MPPT ==
  note: Maximum power point tracking by incremental conductance method + Integral regulator
      | -------------------------------------------------------------------------------------------------------------
      | Maximum power point is obtained when dP/dV=0  where P= V*I
      | -> d(V*I)/dV = I + V*dI/dV = 0
      | -> dI/dV = -I/V
      | The integral regulator minimizes the error (dI/dV + I/V)
      | Regulator output = Duty cycle correction
  note: MPPT Controller
  V_PV : Inport
  I_PV : Inport  Port=2
  on/off : Inport  Port=3
  Add1 : Sum  Inputs=|++
  Add2 : Sum  Inputs=+-
  Add3 : Sum  Inputs=+-
  Compare To Zero : simulink/Logic and Bit Operations/Compare To Zero  relop=~=  OutDataTypeStr=uint8
  Constant : Constant  Value=0
  Constant1 : Constant  Value=0
  Constant2 : Constant  Value=1e-6
  Dead Zone : DeadZone  LowerValue=-0.02  UpperValue=+0.02  SaturateOnIntegerOverflow=on
  Discrete-Time Integrator : DiscreteIntegrator  gainval=1  SampleTime=Ts_Control  LimitOutput=on  UpperSaturationLimit=1  LowerSaturationLimit=-1  ICPrevOutput=DiscIntNeverNeededParam  ICPrevScaledInput=DiscIntNeverNeededParam
  Ki Gain : Gain  Gain=7
  Saturation : Saturate  UpperLimit=inf  LowerLimit=eps
  Switch : Switch  Threshold=0.5
  Switch1 : Switch  Threshold=0.5
  Switch2 : Switch  Criteria=u2 ~= 0
  Unit Delay1 : UnitDelay  SampleTime=Ts_Control  HasFrameUpgradeWarning=on
  Unit Delay2 : UnitDelay  SampleTime=Ts_Control  HasFrameUpgradeWarning=on
  div1 : Product  Inputs=*/  RndMeth=Zero
  div2 : Product  Inputs=*/  RndMeth=Zero
  Delta_D : Outport
  tag scope: I_V_MPPT=global, dI_dV_MPPT=global
  wires:
  V_PV/1 -> Add3/1, Saturation/1, Unit Delay1/1  "V"
  div1/1 -> [dI_dV_MPPT], Add1/1  "dI/dV"
  Constant/1 -> Switch/3
  Switch/1 -> Dead Zone/1
  Unit Delay1/1 -> Add3/2
  Compare To Zero/1 -> Switch2/2
  Switch2/1 -> div1/2
  Constant2/1 -> Switch2/3
  I_PV/1 -> Unit Delay2/1, Add2/1, div2/1  "I"
  Unit Delay2/1 -> Add2/2
  Add3/1 -> Compare To Zero/1, Switch2/1  "dV"
  Add2/1 -> div1/1  "dI"
  Saturation/1 -> div2/2
  div2/1 -> Add1/2, [I_V_MPPT]  "I/V"
  Add1/1 -> Switch/1  "error"
  Dead Zone/1 -> Ki Gain/1
  Constant1/1 -> Switch1/3
  Discrete-Time Integrator/1 -> Switch1/1  "Delta_D"
  Switch1/1 -> Delta_D/1
  on/off/1 -> Switch/2, Switch1/2
  Ki Gain/1 -> Discrete-Time Integrator/1

== system PVarray_Grid_IncCondReg_det/Boost Converter Control (MPPT)/Pulse Generator ==
  D : Inport
  Relational Operator : RelationalOperator  Operator=<=  OutDataTypeStr=boolean  RndMeth=Nearest
  Repeating Sequence : simulink/Sources/Repeating Sequence  rep_seq_t="[0  1/Freq]"  rep_seq_y=[0 1]
  Pulses : Outport
  wires:
  D/1 -> Relational Operator/2
  Relational Operator/1 -> Pulses/1
  Repeating Sequence/1 -> Relational Operator/1

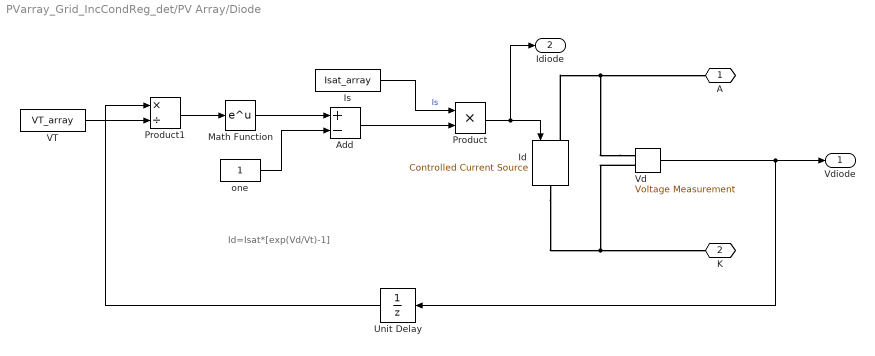
== system PVarray_Grid_IncCondReg_det/PV Array/Diode ==
  note: Id=Isat*[exp(Vd/Vt)-1]
  Add : Sum  Inputs=+-
  Id : powerlib/Electrical Sources/Controlled Current Source  Initialize=on  Source_Type=AC  Amplitude=0  Phase=0  Frequency=0  Measurements=None
      settings: SourceProductName=Simscape Electrical
  Is : Constant  Value=Isat_array
  Math Function : Math  SaturateOnIntegerOverflow=on
  Product : Product  RndMeth=Zero
  Product1 : Product  Inputs=*/  RndMeth=Zero
  Unit Delay : UnitDelay  SampleTime=Ts  HasFrameUpgradeWarning=on
  VT : Constant  Value=VT_array
  Vd : powerlib/Measurements/Voltage Measurement  PhasorSimulation=off  OutputType=Complex  PSBequivalent=0
      settings: SourceProductName=Simscape Electrical
  one : Constant
  A : PMIOPort  Side=Left
  K : PMIOPort  Port=2  Side=Right
  Vdiode : Outport
  Idiode : Outport  Port=2
  wires:
  Product/1 -> Idiode/1, Id/1
  Vd/1 -> Vdiode/1, Unit Delay/1
  Is/1 -> Product/1  "Is"
  Product1/1 -> Math Function/1
  one/1 -> Add/2
  Add/1 -> Product/2
  VT/1 -> Product1/2
  Unit Delay/1 -> Product1/1
  Math Function/1 -> Add/1
  connections:
  Id/RConn1 -- K/RConn1 -- Vd/LConn2
  Vd/LConn1 -- A/RConn1 -- Id/LConn1

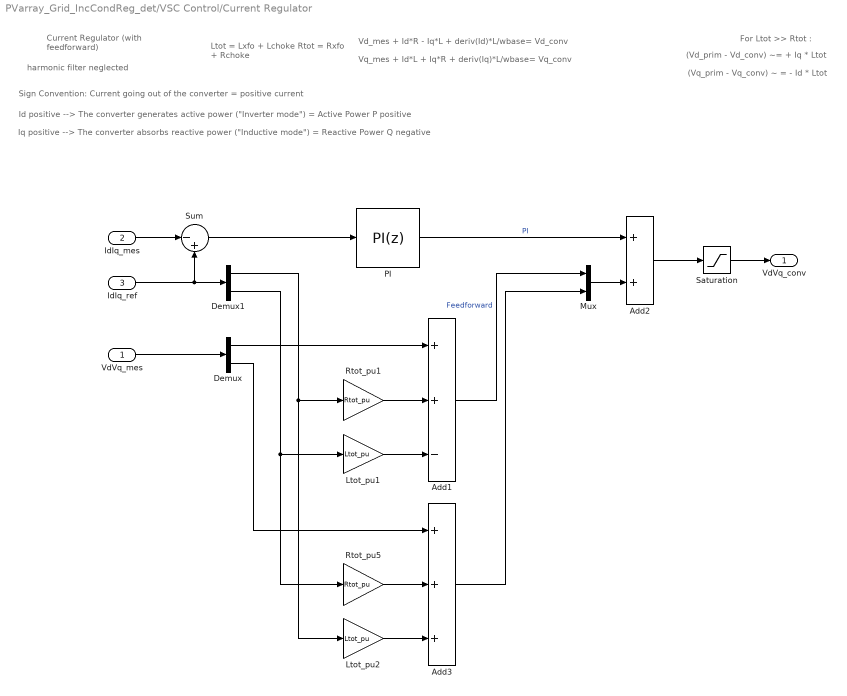
== system PVarray_Grid_IncCondReg_det/VSC Control/Current Regulator ==
  note: harmonic filter neglected
  note: Vd_mes + Id*R - Iq*L + deriv(Id)*L/wbase= Vd_conv
  note: Vq_mes + Id*L + Iq*R + deriv(Iq)*L/wbase= Vq_conv
  note: Current Regulator
      | (with feedforward)
  note: Sign Convention: Current going out of the converter = positive current
  note: Iq positive --> The converter absorbs reactive power ("Inductive mode") = Reactive Power Q negative
  note: Id positive --> The converter generates active power ("Inverter mode") = Active Power P positive
  note: Ltot = Lxfo + Lchoke
      | Rtot = Rxfo + Rchoke
  note: (Vd_prim - Vd_conv) ~= + Iq * Ltot
  note: (Vq_prim - Vq_conv) ~ = - Id * Ltot
  note: For Ltot >> Rtot :
  VdVq_mes : Inport  PortDimensions=2
  IdIq_mes : Inport  Port=2  PortDimensions=2
  IdIq_ref : Inport  Port=3  PortDimensions=2
  Add1 : Sum  Inputs=++-
  Add2 : Sum
  Add3 : Sum  Inputs=+++
  Demux : Demux  Outputs=2
  Demux1 : Demux  Outputs=2
  Ltot_pu1 : Gain  Gain=Ltot_pu  SaturateOnIntegerOverflow=on  OutDataTypeStr=Inherit: Same as input  ParamDataTypeStr=Inherit: Same as input
  Ltot_pu2 : Gain  Gain=Ltot_pu  SaturateOnIntegerOverflow=on  OutDataTypeStr=Inherit: Same as input  ParamDataTypeStr=Inherit: Same as input
  Mux : Mux  Inputs=2
  PI : simulink/Continuous/PID Controller  Controller=PI  Form=Parallel  TimeDomain=Discrete-time  SampleTime=Ts  IntegratorMethod=Forward Euler  FilterMethod=Forward Euler  ControllerParametersSource=internal  P=Kp_Ireg  I=Ki_Ireg  D=0  UseFilter=on  N=100  TunerSelectOption=Transfer Function Based (PID Tuner App)  InitialConditionSource=internal  InitialConditionForIntegrator=0  InitialConditionForFilter=0  DifferentiatorICPrevScaledInput=0  ExternalReset=none  TrackingMode=off  Kt=1  LimitOutput=on  UpperSaturationLimit=2  LowerSaturationLimit=-2  LinearizeAsGain=off  AntiWindupMode=none  Kb=1  POutMin=[]  POutMax=[]  IOutMin=[]  IOutMax=[]  DOutMin=[]  DOutMax=[]  NOutMin=[]  NOutMax=[]  SumOutMin=[]  SumOutMax=[]  SaturationOutMin=[]  SaturationOutMax=[]  PParamMin=[]  PParamMax=[]  IParamMin=[]  IParamMax=[]  DParamMin=[]  DParamMax=[]  NParamMin=[]  NParamMax=[]  KbParamMin=[]  KbParamMax=[]  KtParamMin=[]  KtParamMax=[]  KbOutMin=[]  KbOutMax=[]  KtOutMin=[]  KtOutMax=[]  IntegratorOutMin=[]  IntegratorOutMax=[]  FilterOutMin=[]  FilterOutMax=[]  SumI1OutMin=[]  SumI1OutMax=[]  SumI2OutMin=[]  SumI2OutMax=[]  SumI3OutMin=[]  SumI3OutMax=[]  SumI4OutMin=[]  SumI4OutMax=[]  SumDOutMin=[]  SumDOutMax=[]  DifferentiatorOutMin=[]  DifferentiatorOutMax=[]  FilterDiffOutCoefMin=[]  FilterDiffOutCoefMax=[]  ReciprocalOutMin=[]  ReciprocalOutMax=[]  SumDenOutMin=[]  SumDenOutMax=[]  SumNumOutMin=[]  SumNumOutMax=[]  DivideOutMin=[]  DivideOutMax=[]  IntegratorContinuousStateAttributes=''  IntegratorStateMustResolveToSignalObject=off  IntegratorRTWStateStorageClass=Auto  FilterContinuousStateAttributes=''  FilterStateMustResolveToSignalObject=off  FilterRTWStateStorageClass=Auto  ParallelPVariant=InternalParameters  IdealPVariant=Disabled  IVariant=InternalParameters  DVariant=Disabled  IntegratorVariant=Discrete  SatVariant=Enabled  AWVariant=Passthrough  PCopyVariant=Disabled  TRVariant=Disabled  FdbkBlocksVariant=Forward  IdealPFdbkVariant=Disabled  SatFdbkVariant=Disabled  DerivativeFilterVariant=Disabled  NVariant=Disabled  NCopyVariant=Disabled_SignalSpec  FilterICVariant=Disabled  IntegratorICVariant=InternalICs  ExternalResetVariant=Disabled  TRSumVariant=Passthrough  SumFdbkVariant=Disabled  SumVariant=Sum_PI
  Rtot_pu1 : Gain  Gain=Rtot_pu  SaturateOnIntegerOverflow=on  OutDataTypeStr=Inherit: Same as input  ParamDataTypeStr=Inherit: Same as input
  Rtot_pu5 : Gain  Gain=Rtot_pu  SaturateOnIntegerOverflow=on  OutDataTypeStr=Inherit: Same as input  ParamDataTypeStr=Inherit: Same as input
  Saturation : Saturate  UpperLimit=2  LowerLimit=-2
  Sum : Sum  Inputs=|-+
  VdVq_conv : Outport
  wires:
  Mux/1 -> Add2/2
  PI/1 -> Add2/1  "PI"
  Sum/1 -> PI/1
  IdIq_ref/1 -> Sum/2, Demux1/1
  IdIq_mes/1 -> Sum/1
  Add2/1 -> Saturation/1
  Saturation/1 -> VdVq_conv/1
  VdVq_mes/1 -> Demux/1
  Demux/1 -> Add1/1
  Rtot_pu1/1 -> Add1/2
  Demux1/1 -> Rtot_pu1/1, Ltot_pu2/1
  Ltot_pu1/1 -> Add1/3
  Demux1/2 -> Ltot_pu1/1, Rtot_pu5/1
  Rtot_pu5/1 -> Add3/2
  Ltot_pu2/1 -> Add3/3
  Add1/1 -> Mux/1  "Feedforward"
  Demux/2 -> Add3/1
  Add3/1 -> Mux/2

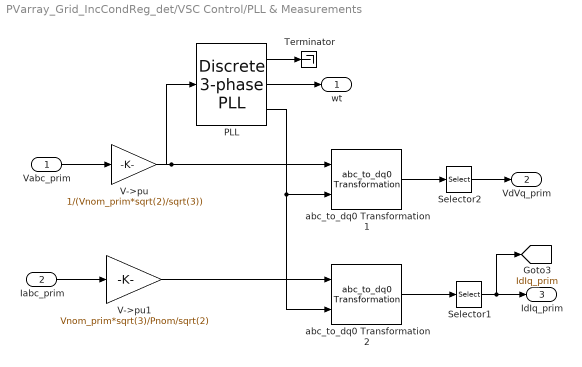
== system PVarray_Grid_IncCondReg_det/VSC Control/PLL & Measurements ==
  Vabc_prim : Inport
  Iabc_prim : Inport  Port=2
  PLL : powerlib_extras/Discrete  Control Blocks/Discrete 3-phase PLL  Fmin=45  Par_Init="[-0.57  Fnom]"  ParK=[60 1400]  Ts=Ts  AGC=off
      settings: SourceProductName=Simscape Electrical  SourceProductBaseCode=PS
  Selector1 : Selector  InputPortWidth=3  IndexOptions=Index vector (dialog)  Indices=[1 2]  OutputSizes=1
  Selector2 : Selector  InputPortWidth=3  IndexOptions=Index vector (dialog)  Indices=[1 2]  OutputSizes=1
  Terminator : Terminator
  V->pu : Gain  Gain=1/(Vnom_prim*sqrt(2)/sqrt(3))  SaturateOnIntegerOverflow=on  OutDataTypeStr=Inherit: Same as input  ParamDataTypeStr=Inherit: Same as input
  V->pu1 : Gain  Gain=Vnom_prim*sqrt(3)/Pnom/sqrt(2)  SaturateOnIntegerOverflow=on  OutDataTypeStr=Inherit: Same as input  ParamDataTypeStr=Inherit: Same as input
  abc_to_dq0 Transformation1 : powerlib_extras/Measurements/abc_to_dq0 Transformation
      settings: SourceProductName=Simscape Electrical  SourceProductBaseCode=PS
  abc_to_dq0 Transformation2 : powerlib_extras/Measurements/abc_to_dq0 Transformation
      settings: SourceProductName=Simscape Electrical  SourceProductBaseCode=PS
  wt : Outport
  VdVq_prim : Outport  Port=2
  IdIq_prim : Outport  Port=3
  tag scope: IdIq_prim=global
  wires:
  V->pu1/1 -> abc_to_dq0 Transformation2/1
  V->pu/1 -> PLL/1, abc_to_dq0 Transformation1/1
  abc_to_dq0 Transformation2/1 -> Selector1/1
  PLL/2 -> wt/1
  Vabc_prim/1 -> V->pu/1
  Iabc_prim/1 -> V->pu1/1
  abc_to_dq0 Transformation1/1 -> Selector2/1
  Selector2/1 -> VdVq_prim/1
  Selector1/1 -> [IdIq_prim], IdIq_prim/1
  PLL/3 -> abc_to_dq0 Transformation2/2, abc_to_dq0 Transformation1/2
  PLL/1 -> Terminator/1

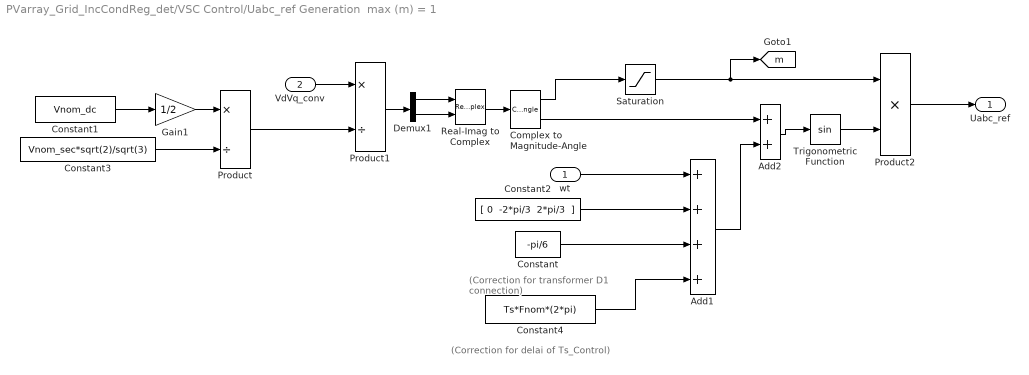
== system PVarray_Grid_IncCondReg_det/VSC Control/Uabc_ref Generation  max (m) = 1 ==
  note: (Correction for transformer
      |  D1 connection)
  note: (Correction for delai of Ts_Control)
  wt : Inport
  VdVq_conv : Inport  Port=2
  Add1 : Sum  Inputs=++++
  Add2 : Sum
  Complex to Magnitude-Angle : ComplexToMagnitudeAngle
  Constant : Constant  Value=-pi/6
  Constant1 : Constant  Value=Vnom_dc
  Constant2 : Constant  Value="[ 0  -2*pi/3  2*pi/3  ]"
  Constant3 : Constant  Value=Vnom_sec*sqrt(2)/sqrt(3)
  Constant4 : Constant  Value=Ts*Fnom*(2*pi)
  Demux1 : Demux  Outputs=2
  Gain1 : Gain  Gain=1/2
  Product : Product  Inputs=*/  RndMeth=Zero
  Product1 : Product  Inputs=*/  RndMeth=Zero
  Product2 : Product  Inputs=**  RndMeth=Zero
  Real-Imag to Complex : RealImagToComplex
  Saturation : Saturate  UpperLimit=1  LowerLimit=0
  Trigonometric Function : Trigonometry
  Uabc_ref : Outport
  tag scope: m=global
  wires:
  Complex to Magnitude-Angle/1 -> Saturation/1
  Constant1/1 -> Gain1/1
  VdVq_conv/1 -> Product1/1
  Product1/1 -> Demux1/1
  Gain1/1 -> Product/1
  Real-Imag to Complex/1 -> Complex to Magnitude-Angle/1
  Demux1/1 -> Real-Imag to Complex/1
  Demux1/2 -> Real-Imag to Complex/2
  Constant2/1 -> Add1/2
  Constant/1 -> Add1/3
  Constant3/1 -> Product/2
  Product/1 -> Product1/2
  Complex to Magnitude-Angle/2 -> Add2/1
  Add1/1 -> Add2/2
  Add2/1 -> Trigonometric Function/1
  Saturation/1 -> [m], Product2/1
  Trigonometric Function/1 -> Product2/2
  Product2/1 -> Uabc_ref/1
  wt/1 -> Add1/1
  Constant4/1 -> Add1/4

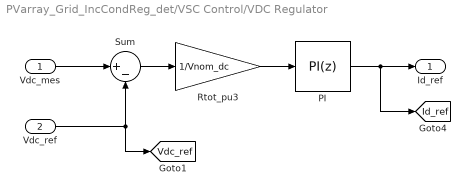
== system PVarray_Grid_IncCondReg_det/VSC Control/VDC Regulator ==
  Vdc_mes : Inport  PortDimensions=1
  Vdc_ref : Inport  Port=2  PortDimensions=1
  PI : simulink/Continuous/PID Controller  Controller=PI  Form=Parallel  TimeDomain=Discrete-time  SampleTime=Ts  IntegratorMethod=Trapezoidal  FilterMethod=Forward Euler  ControllerParametersSource=internal  P=Kp_VDCreg  I=Ki_VDCreg  D=0  UseFilter=on  N=100  TunerSelectOption=Transfer Function Based (PID Tuner App)  InitialConditionSource=internal  InitialConditionForIntegrator=0  InitialConditionForFilter=0  DifferentiatorICPrevScaledInput=0  ExternalReset=none  TrackingMode=off  Kt=1  LimitOutput=on  UpperSaturationLimit=1.5  LowerSaturationLimit=-1.5  LinearizeAsGain=off  AntiWindupMode=none  Kb=1  POutMin=[]  POutMax=[]  IOutMin=[]  IOutMax=[]  DOutMin=[]  DOutMax=[]  NOutMin=[]  NOutMax=[]  SumOutMin=[]  SumOutMax=[]  SaturationOutMin=[]  SaturationOutMax=[]  PParamMin=[]  PParamMax=[]  IParamMin=[]  IParamMax=[]  DParamMin=[]  DParamMax=[]  NParamMin=[]  NParamMax=[]  KbParamMin=[]  KbParamMax=[]  KtParamMin=[]  KtParamMax=[]  KbOutMin=[]  KbOutMax=[]  KtOutMin=[]  KtOutMax=[]  IntegratorOutMin=[]  IntegratorOutMax=[]  FilterOutMin=[]  FilterOutMax=[]  SumI1OutMin=[]  SumI1OutMax=[]  SumI2OutMin=[]  SumI2OutMax=[]  SumI3OutMin=[]  SumI3OutMax=[]  SumI4OutMin=[]  SumI4OutMax=[]  SumDOutMin=[]  SumDOutMax=[]  DifferentiatorOutMin=[]  DifferentiatorOutMax=[]  FilterDiffOutCoefMin=[]  FilterDiffOutCoefMax=[]  ReciprocalOutMin=[]  ReciprocalOutMax=[]  SumDenOutMin=[]  SumDenOutMax=[]  SumNumOutMin=[]  SumNumOutMax=[]  DivideOutMin=[]  DivideOutMax=[]  IntegratorContinuousStateAttributes=''  IntegratorStateMustResolveToSignalObject=off  IntegratorRTWStateStorageClass=Auto  FilterContinuousStateAttributes=''  FilterStateMustResolveToSignalObject=off  FilterRTWStateStorageClass=Auto  ParallelPVariant=InternalParameters  IdealPVariant=Disabled  IVariant=InternalParameters  DVariant=Disabled  IntegratorVariant=Discrete  SatVariant=Enabled  AWVariant=Passthrough  PCopyVariant=Disabled  TRVariant=Disabled  FdbkBlocksVariant=Forward  IdealPFdbkVariant=Disabled  SatFdbkVariant=Disabled  DerivativeFilterVariant=Disabled  NVariant=Disabled  NCopyVariant=Disabled_SignalSpec  FilterICVariant=Disabled  IntegratorICVariant=InternalICs  ExternalResetVariant=Disabled  TRSumVariant=Passthrough  SumFdbkVariant=Disabled  SumVariant=Sum_PI
  Rtot_pu3 : Gain  Gain=1/Vnom_dc  SaturateOnIntegerOverflow=on  OutDataTypeStr=Inherit: Same as input  ParamDataTypeStr=Inherit: Same as input
  Sum : Sum  Inputs=|+-
  Id_ref : Outport  SampleTime=Ts  InitialOutput=0
  tag scope: Id_ref=global, Vdc_ref=global
  wires:
  Sum/1 -> Rtot_pu3/1
  Vdc_mes/1 -> Sum/1
  Vdc_ref/1 -> Sum/2, [Vdc_ref]
  Rtot_pu3/1 -> PI/1
  PI/1 -> [Id_ref], Id_ref/1
